simulink model "latLongOkay"  (R2018b)
settings: Solver=VariableStepAuto  StartTime=0.0  StopTime=10.0  RelTol=1e-3
libraries: robotlib x3
settings Model: Creator=haari  LastModifiedBy=KaSat

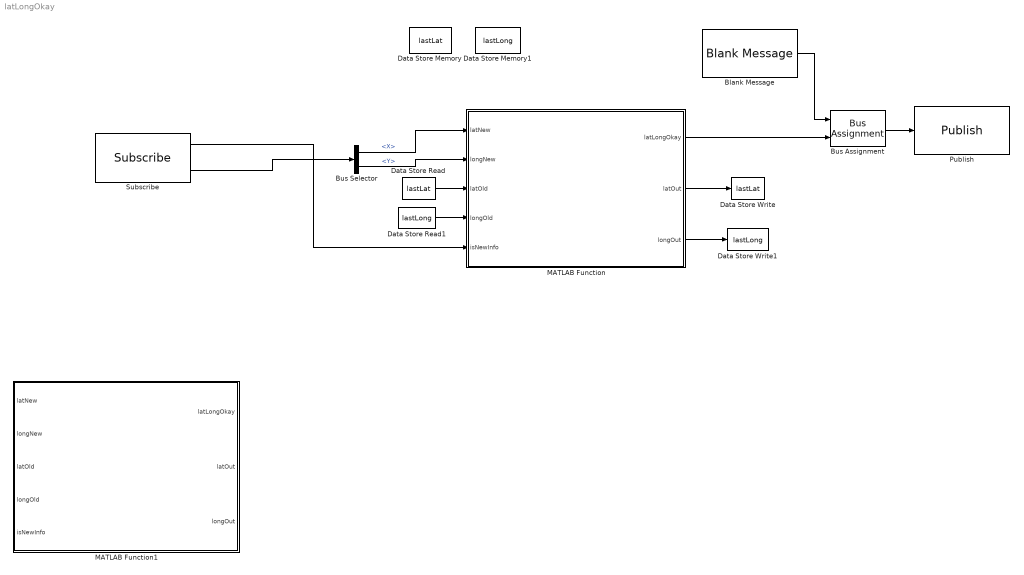
== system latLongOkay ==
  Blank Message : robotlib/Blank Message  messageClass=Message  entityType=std_msgs/Bool  messageType=std_msgs/Bool  SampleTime=inf
      settings: SourceProductBaseCode=RO
  Bus Assignment : BusAssignment  AssignedSignals=Data
  Bus Selector : BusSelector  OutputSignals=X,Y
  Data Store Memory : DataStoreMemory  DataStoreName=lastLat  ReadBeforeWriteMsg=warning  WriteAfterWriteMsg=warning  WriteAfterReadMsg=warning  ShowAdditionalParam=off
  Data Store Memory1 : DataStoreMemory  DataStoreName=lastLong  ReadBeforeWriteMsg=warning  WriteAfterWriteMsg=warning  WriteAfterReadMsg=warning  ShowAdditionalParam=off
  Data Store Read : DataStoreRead  DataStoreName=lastLat
  Data Store Read1 : DataStoreRead  DataStoreName=lastLong
  Data Store Write : DataStoreWrite  DataStoreName=lastLat
  Data Store Write1 : DataStoreWrite  DataStoreName=lastLong
  MATLAB Function : MATLAB Function  TreatAsAtomicUnit=on
  MATLAB Function1 : MATLAB Function  TreatAsAtomicUnit=on
  Publish : robotlib/Publish  topicSource=Specify your own  topic=/latlongflag  messageType=std_msgs/Bool  messageQueueLength=1
      settings: SourceProductBaseCode=RO
  Subscribe : robotlib/Subscribe  topicSource=Specify your own  topic=/location  messageType=geometry_msgs/Point  sampleTime=-1  messageQueueLength=1
      settings: SourceProductBaseCode=RO
  wires:
  Subscribe/2 -> Bus Selector/1
  Bus Selector/1 -> MATLAB Function/1(latNew)  "<X>"
  Bus Selector/2 -> MATLAB Function/2(longNew)  "<Y>"
  Subscribe/1 -> MATLAB Function/5(isNewInfo)
  Data Store Read/1 -> MATLAB Function/3(latOld)
  MATLAB Function/2(latOut) -> Data Store Write/1
  Data Store Read1/1 -> MATLAB Function/4(longOld)
  MATLAB Function/3(longOut) -> Data Store Write1/1
  Bus Assignment/1 -> Publish/1
  Blank Message/1 -> Bus Assignment/1
  MATLAB Function/1(latLongOkay) -> Bus Assignment/2

== matlab function latLongOkay/MATLAB Function1 ==
  data: latNew input; latLongOkay output; longNew input; latOld input; longOld input; isNewInfo input; latOut output; longOut output
function [latLongOkay, latOut, longOut] = fcn(latNew, longNew, latOld, longOld ,isNewInfo)
%Return old data if not new data
if isNewInfo == false
    latLongOkay = true;
    latOut = latOld;
    longOut = longOld;
    return;
end

%Check if lat and long zero
if (latNew == 0) || (longNew == 0)
    latLongOkay = false;
    latOut = latOld;
    longOut = longOld;
    return;
end

%Check if change too large (20m)
%Uses Haversine function from online file exchange
radius=6371;
lat1=latNew*pi/180;
lat2=latOld*pi/180;
lon1=longNew*pi/180;
lon2=longOld*pi/180;
deltaLat=lat2-lat1;
deltaLon=lon2-lon1;
a=sin((deltaLat)/2)^2 + cos(lat1)*cos(lat2) * sin(deltaLon/2)^2;
c=2*atan2(sqrt(a),sqrt(1-a));
dist=(radius*c)/1000;    %Haversine distance in meters

if dist>20
    latLongOkay = false;
    latOut = latNew;
    longOut = longNew;
end

%else return new data
latOut = latNew;
longOut = longNew;
latLongOkay = true;
end

== matlab function latLongOkay/MATLAB Function ==
  data: latNew input; latLongOkay output; longNew input; latOld input; longOld input; isNewInfo input; latOut output; longOut output
function [latLongOkay, latOut, longOut] = fcn(latNew, longNew, latOld, longOld ,isNewInfo)
%Return old data if not new data
if isNewInfo == false
    latLongOkay = true;
    latOut = latOld;
    longOut = longOld;
    return;
end

%Check if lat and long zero
if (latNew == 0) || (longNew == 0)
    latLongOkay = false;
    latOut = latOld;
    longOut = longOld;
    return;
end

%Check if change too large (20m)
%Uses Haversine function from online file exchange
radius=6371;
lat1=latNew*pi/180;
lat2=latOld*pi/180;
lon1=longNew*pi/180;
lon2=longOld*pi/180;
deltaLat=lat2-lat1;
deltaLon=lon2-lon1;
a=sin((deltaLat)/2)^2 + cos(lat1)*cos(lat2) * sin(deltaLon/2)^2;
c=2*atan2(sqrt(a),sqrt(1-a));
dist=(radius*c)/1000;    %Haversine distance in meters

if dist>20
    latLongOkay = false;
    latOut = latNew;
    longOut = longNew;
end

%else return new data
latOut = latNew;
longOut = longNew;
latLongOkay = true;
end
